simulink model "w2p3"  (R2020b)
settings: Solver=ode45  StartTime=0.0  StopTime=120  RelTol=1e-3
model workspace (MAT data in the model file):
  Ki = 150
  Kp = 90
  Sig = Simulink.Signal
  Sig.DataType = 'auto'
  Sig.Dimensions = -1
  Sig.DimensionsMode = 'auto'
  Sig.Complexity = 'auto'
  Sig.SampleTime = -1
  Sig.SamplingMode = 'auto'
  Ts = 0.01
  b = 50
  m = 1000
settings Model: DataDictionary=prob3_Cruise_Control.sldd  Creator=Rasika Shejul  LastModifiedBy=family

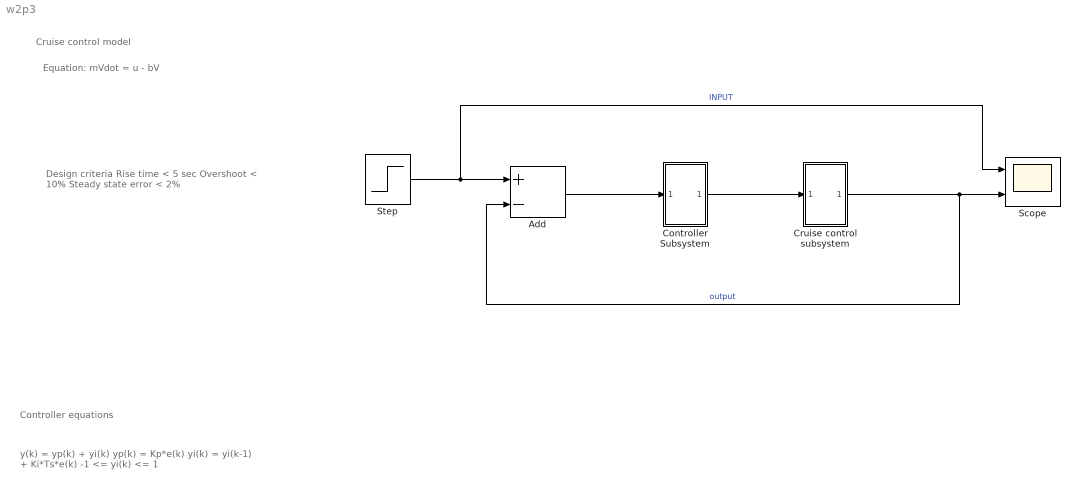
== system w2p3 ==
  note: Design criteria
      | Rise time < 5 sec
      | Overshoot < 10%
      | Steady state error < 2%
  note: Controller equations
  note: y(k) = yp(k) + yi(k)
      | yp(k) = Kp*e(k)
      | yi(k) = yi(k-1) + Ki*Ts*e(k)
      | -1 <= yi(k) <= 1
  note: Equation:
      | mVdot = u - bV
  note: Cruise control model
  Add : Sum  Inputs=+-
  Controller Subsystem : Subsystem
  Cruise control subsystem : Subsystem
  Scope : Scope  NumInputPorts=2
  Step : Step  SampleTime=0
  wires:
  Add/1 -> Controller Subsystem/1(In1)
  Controller Subsystem/1(Output) -> Cruise control subsystem/1(Inport)
  Cruise control subsystem/1(Output) -> Add/2, Scope/2  "output"
  Step/1 -> Scope/1, Add/1  "INPUT"

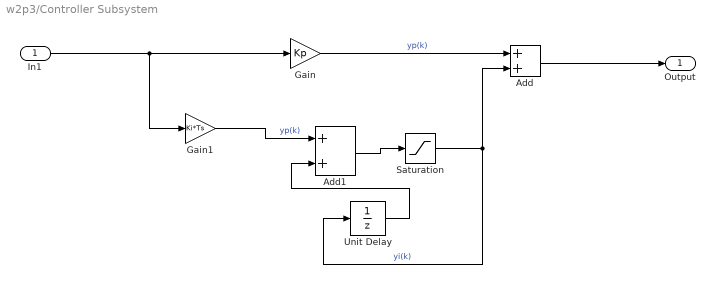
== system w2p3/Controller Subsystem ==
  In1 : Inport
  Add : Sum
  Add1 : Sum
  Gain : Gain  Gain=Kp
  Gain1 : Gain  Gain=Ki*Ts
  Saturation : Saturate  UpperLimit=1  LowerLimit=-1
  Unit Delay : UnitDelay  SampleTime=-1  HasFrameUpgradeWarning=on
  Output : Outport
  wires:
  In1/1 -> Gain1/1, Gain/1
  Gain1/1 -> Add1/1  "yp(k)"
  Unit Delay/1 -> Add1/2
  Add/1 -> Output/1
  Gain/1 -> Add/1  "yp(k)"
  Saturation/1 -> Add/2, Unit Delay/1  "yi(k)"
  Add1/1 -> Saturation/1

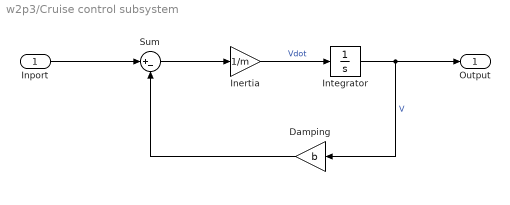
== system w2p3/Cruise control subsystem ==
  Inport : Inport
  Damping : Gain  Gain=b
  Inertia : Gain  Gain=1/m
  Integrator : Integrator
  Sum : Sum  Inputs=|+-
  Output : Outport
  wires:
  Inport/1 -> Sum/1
  Inertia/1 -> Integrator/1  "Vdot"
  Integrator/1 -> Output/1, Damping/1  "V"
  Damping/1 -> Sum/2
  Sum/1 -> Inertia/1
